simulink model "PistonControllerOff"  (R2013a)
settings: Solver=FixedStepDiscrete  StartTime=0.0  StopTime=75  FixedStep=0.001  RelTol=1e-3
InitFcn:
  | % PI gains
  | 
  | P1 = 15.0;
  | I1 = 100.0;
  | D1 = 10.0;
  | N1 = 10;
  | 
  | 
  | P2 =15.0 ;
  | I2 = 100.0;
  | D2 = 0.0;
  | N2 = 5;
  | 
  | P3 = 15.0;
  | I3 = 100.0;
  | D3 = 0.0;
  | N3 = 5;
  | 
  | P4 =15.0;
  | I4 = 100.0;
  | D4 =0.0;
  | N4 = 5;
  | 
  | P5 = 15.0;
  | I5 = 100.0;
  | D5 = 0.0;
  | N5 = 5;
  | 
  | P6 = 40.0;
  | I6 = 100.0;
  | D6 = 0.0;
  | N6 = 5.0;
  | 
  | P7 = 6.7;
  | I7 = 0.0;
  | D7 = 0.0;
  | N7 = 10.0;
  | 
  | %Max = Left = positive
  | 
  | offset = 1000;
  | 
  | max1 = 2300;
  | min1 = -2300;
  | 
  | max2 = 2500;
  | min2 = -2500;
  | 
  | max3 = 2600;
  | min3 = -2600;
  | 
  | max4 = 2600;
  | min4 = -2600;
  | 
  | max5 = 2600;
  | min5 = -2600;
  | 
  | max6 = 2400;
  | min6 = -2400;
  | 
  | 
  | max_posG = 1800;
undefined symbols (not defined in the file or in its folder): rtwindemocb_modeswitch, Serial_Port, Standard_Devices
libraries: rtwinlib x14, simulink x7
Description:
  | Packet Input/Output
  | 
  | This model shows how to transfer data through UDP
  | communication protocol using binary encoding. The model sends data
  | within one computer, from one UDP port to another. You can modify the
  | model to communicate between two computers by splitting this model
  | into its send and receive parts and running the models on two computers.
  | The yellow blocks are used to send the data, the blue blocks
  | are used to receive the data. Then, please enter the IP addresses of the two
  | computers into the appropriate fields in the Board Setup dialog.
  | 
  | How to run this model in Normal Mode:
  | 
  | 1) Double-click the orange button to switch to Normal Mode if needed.
  | 2) Start the real-time execution using Simulation->Run.
  | 
  | How to run this model in External Mode:
  | 
  | 1) Double-click the orange button to switch to External Mode if needed.
  | 2) Build the model using Code->C/C++ Code->Build Model.
  | 3) Connect to the real-time code using Simulation->Connect To Target.
  | 4) Start the real-time execution using Simulation->Run.
settings Model: SimulationMode=external  ExtModeTrigDuration=75001  Creator=The MathWorks Inc.  LastModifiedBy=drl
settings DataIOCC: SignalLoggingSaveFormat=ModelDataLogs
settings OptimizationCC: InlineParams=on  InlineInvariantSignals=on  EnhancedBackFolding=on  ExpressionDepthLimit=2147483647  InitFltsAndDblsToZero=on  EfficientFloat2IntCast=on  EfficientMapNaN2IntZero=off  SimCompilerOptimization=On
settings DebuggingCC: MultiTaskDSMMsg=warning  MultiTaskCondExecSysMsg=none  FcnCallInpInsideContextMsg=EnableAllAsWarning  StrictBusMsg=None
settings HardwareCC: ProdIntDivRoundTo=Zero  ProdEndianess=LittleEndian  ProdHWDeviceType=32-bit Real-Time Windows Target  TargetIntDivRoundTo=Zero  TargetEndianess=LittleEndian  TargetHWDeviceType=32-bit Real-Time Windows Target
settings ModelReferenceCC: UpdateModelReferenceTargets=IfOutOfDate
settings SFSimCC: SFSimEcho=off
settings RTWCC: SystemTargetFile=rtwin.tlc  TemplateMakefile=rtwin.tmf  Description=Real-Time Windows Target  ProcessScript=rtwin_make_rtw_hook  IncludeERTFirstTime=on  RTWCompilerOptimization=On
settings RTWinTargetCC: TargetLibSuffix=_rtwin.lib  TargetPreCompLibLocation=C:\Program Files\MATLAB\R2013a\toolbox\rtw\targets\rtwin\lib\win64  CodeReplacementLibrary=ANSI_C  RTWinDir=C:/PROGRA~1/MATLAB/R2013a/toolbox/rtw/targets/rtwin  TargetArch=win64

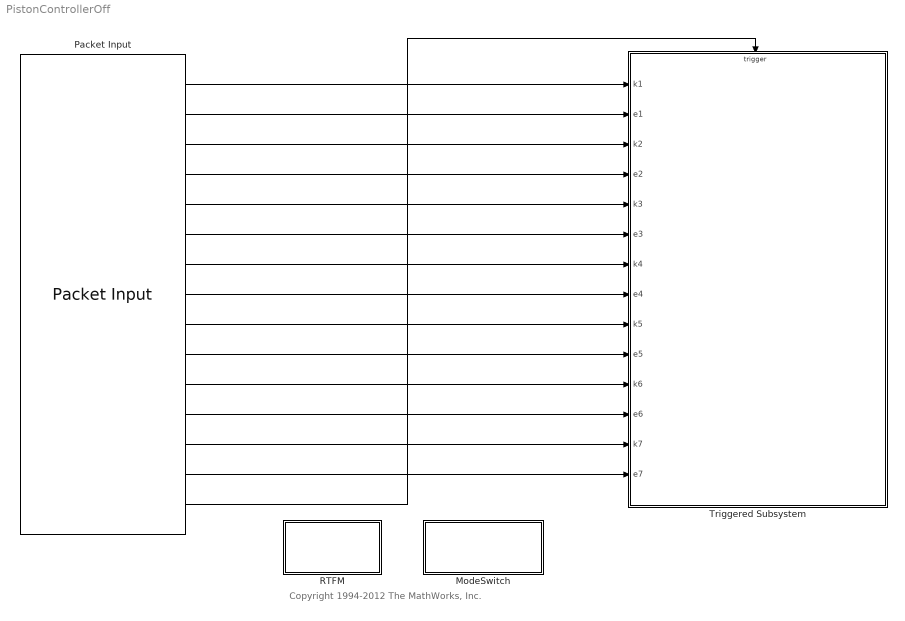
== system PistonControllerOff ==
  note: Copyright 1994-2012 The MathWorks, Inc.
  ModeSwitch : Subsystem  InitFcn=rtwindemocb_modeswitch('CheckKernel');  mask(Real-Time Windows Target Example Mode Switch){}
      settings: OpenFcn=rtwindemocb_modeswitch(gcbh);
      mask Display: disp('Switch To\nNormal Mode');
  Packet Input : rtwinlib/Packet Input  SampleTime=0.001  MaxMissedTicks=10000  ShowMissedTicks=off  YieldWhenWaiting=off  DrvName=Standard_Devices/Serial_Port  DrvAddress=39  DrvOptions=[57600 8 0 0 0 0 0 0]  PacketSize=14  DataTypes={'int8','int8','int8','int8','int8','int8','int8','int8','int8','int8','int8','int8','int8','int8'}  ShowReady=on  ShowError=off  PacketID=1  ByteOrder=1  ShowTimestamp=off
      settings: AttributesFormatString=Standard Devices\nSerial Port [27h]
  "RTFM " : Subsystem  mask(Real-Time Windows Target Example Info){}
      settings: OpenFcn=web(fullfile(fileparts(which(gcs)), 'html', [gcs '.html']), '-helpbrowser');
      mask Display: disp('Info')
  Triggered Subsystem : Subsystem  TreatAsAtomicUnit=on
  wires:
  Packet Input/10 -> Triggered Subsystem/10(e5)
  Packet Input/4 -> Triggered Subsystem/4(e2)
  Packet Input/12 -> Triggered Subsystem/12(e6)
  Packet Input/8 -> Triggered Subsystem/8(e4)
  Packet Input/9 -> Triggered Subsystem/9(k5)
  Packet Input/11 -> Triggered Subsystem/11(k6)
  Packet Input/5 -> Triggered Subsystem/5(k3)
  Packet Input/7 -> Triggered Subsystem/7(k4)
  Packet Input/6 -> Triggered Subsystem/6(e3)
  Packet Input/1 -> Triggered Subsystem/1(k1)
  Packet Input/3 -> Triggered Subsystem/3(k2)
  Packet Input/2 -> Triggered Subsystem/2(e1)
  Packet Input/13 -> Triggered Subsystem/13(k7)
  Packet Input/14 -> Triggered Subsystem/14(e7)
  Packet Input/15 -> Triggered Subsystem/Trigger

== system PistonControllerOff/ModeSwitch ==

== system PistonControllerOff/RTFM  ==

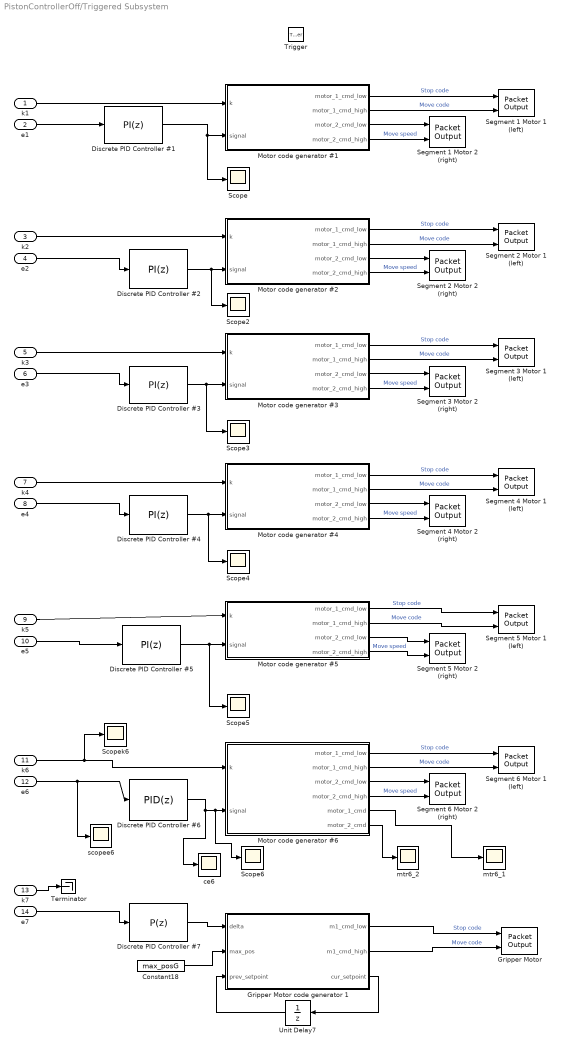
== system PistonControllerOff/Triggered Subsystem ==
  k1 : Inport
  e1 : Inport  Port=2
  k2 : Inport  Port=3
  e2 : Inport  Port=4
  k3 : Inport  Port=5
  e3 : Inport  Port=6
  k4 : Inport  Port=7
  e4 : Inport  Port=8
  k5 : Inport  Port=9
  e5 : Inport  Port=10
  k6 : Inport  Port=11
  e6 : Inport  Port=12
  k7 : Inport  Port=13
  e7 : Inport  Port=14
  Trigger : TriggerPort
  Constant18 : Constant  Value=max_posG
  Discrete PID Controller #1 : simulink/Continuous/PID Controller  Controller=PI  TimeDomain=Discrete-time  SampleTime=-1  IntegratorMethod=Forward Euler  FilterMethod=Forward Euler  Form=Parallel  P=P1  I=I1  D=D1  N=N1  InitialConditionSource=internal  InitialConditionForIntegrator=0  InitialConditionForFilter=0  ExternalReset=none  LimitOutput=on  UpperSaturationLimit=max1  LowerSaturationLimit=min1  LinearizeAsGain=off  AntiWindupMode=clamping  Kb=1  TrackingMode=off  Kt=10  RndMeth=Nearest  SaturateOnIntegerOverflow=on  PParamMin=[]  PParamMax=[]  PParamDataTypeStr=double  IParamMin=[]  IParamMax=[]  IParamDataTypeStr=double  DParamMin=[]  DParamMax=[]  DParamDataTypeStr=double  NParamMin=[]  NParamMax=[]  NParamDataTypeStr=double  KbParamMin=[]  KbParamMax=[]  KtParamMin=[]  KtParamMax=[]  KtParamDataTypeStr=double  POutMin=[]  POutMax=[]  POutDataTypeStr=double  IOutMin=[]  IOutMax=[]  IOutDataTypeStr=double  DOutMin=[]  DOutMax=[]  DOutDataTypeStr=double  NOutMin=[]  NOutMax=[]  NOutDataTypeStr=double  KbOutMin=[]  KbOutMax=[]  KtOutMin=[]  KtOutMax=[]  KtOutDataTypeStr=double  IntegratorOutMin=[]  IntegratorOutMax=[]  IntegratorOutDataTypeStr=double  FilterOutMin=[]  FilterOutMax=[]  FilterOutDataTypeStr=double  SumOutMin=[]  SumOutMax=[]  SumOutDataTypeStr=double  SumI1OutMin=[]  SumI1OutMax=[]  SumI1OutDataTypeStr=double  SumI2OutMin=[]  SumI2OutMax=[]  SumI3OutMin=[]  SumI3OutMax=[]  SumI3OutDataTypeStr=double  SumDOutMin=[]  SumDOutMax=[]  SumDOutDataTypeStr=double  SumAccumDataTypeStr=double  SumI1AccumDataTypeStr=double  SumI3AccumDataTypeStr=double  SumDAccumDataTypeStr=double  SaturationOutMin=[]  SaturationOutMax=[]  SaturationOutDataTypeStr=double  IntegratorContinuousStateAttributes=''  IntegratorStateMustResolveToSignalObject=off  IntegratorRTWStateStorageClass=Auto  FilterContinuousStateAttributes=''  FilterStateMustResolveToSignalObject=off  FilterRTWStateStorageClass=Auto
  Discrete PID Controller #2 : simulink/Continuous/PID Controller  Controller=PI  TimeDomain=Discrete-time  SampleTime=-1  IntegratorMethod=Forward Euler  FilterMethod=Forward Euler  Form=Parallel  P=P2  I=I2  D=D2  N=N2  InitialConditionSource=internal  InitialConditionForIntegrator=0  InitialConditionForFilter=0  ExternalReset=none  LimitOutput=on  UpperSaturationLimit=max2  LowerSaturationLimit=min2  LinearizeAsGain=off  AntiWindupMode=clamping  Kb=1  TrackingMode=off  Kt=10  RndMeth=Nearest  SaturateOnIntegerOverflow=on  PParamMin=[]  PParamMax=[]  PParamDataTypeStr=double  IParamMin=[]  IParamMax=[]  IParamDataTypeStr=double  DParamMin=[]  DParamMax=[]  DParamDataTypeStr=double  NParamMin=[]  NParamMax=[]  NParamDataTypeStr=double  KbParamMin=[]  KbParamMax=[]  KtParamMin=[]  KtParamMax=[]  KtParamDataTypeStr=double  POutMin=[]  POutMax=[]  POutDataTypeStr=double  IOutMin=[]  IOutMax=[]  IOutDataTypeStr=double  DOutMin=[]  DOutMax=[]  DOutDataTypeStr=double  NOutMin=[]  NOutMax=[]  NOutDataTypeStr=double  KbOutMin=[]  KbOutMax=[]  KtOutMin=[]  KtOutMax=[]  KtOutDataTypeStr=double  IntegratorOutMin=[]  IntegratorOutMax=[]  IntegratorOutDataTypeStr=double  FilterOutMin=[]  FilterOutMax=[]  FilterOutDataTypeStr=double  SumOutMin=[]  SumOutMax=[]  SumOutDataTypeStr=double  SumI1OutMin=[]  SumI1OutMax=[]  SumI1OutDataTypeStr=double  SumI2OutMin=[]  SumI2OutMax=[]  SumI3OutMin=[]  SumI3OutMax=[]  SumI3OutDataTypeStr=double  SumDOutMin=[]  SumDOutMax=[]  SumDOutDataTypeStr=double  SumAccumDataTypeStr=double  SumI1AccumDataTypeStr=double  SumI3AccumDataTypeStr=double  SumDAccumDataTypeStr=double  SaturationOutMin=[]  SaturationOutMax=[]  SaturationOutDataTypeStr=double  IntegratorContinuousStateAttributes=''  IntegratorStateMustResolveToSignalObject=off  IntegratorRTWStateStorageClass=Auto  FilterContinuousStateAttributes=''  FilterStateMustResolveToSignalObject=off  FilterRTWStateStorageClass=Auto
  Discrete PID Controller #3 : simulink/Continuous/PID Controller  Controller=PI  TimeDomain=Discrete-time  SampleTime=-1  IntegratorMethod=Forward Euler  FilterMethod=Forward Euler  Form=Parallel  P=P3  I=I3  D=D3  N=N3  InitialConditionSource=internal  InitialConditionForIntegrator=0  InitialConditionForFilter=0  ExternalReset=none  LimitOutput=on  UpperSaturationLimit=max3  LowerSaturationLimit=min3  LinearizeAsGain=off  AntiWindupMode=clamping  Kb=1  TrackingMode=off  Kt=10  RndMeth=Nearest  SaturateOnIntegerOverflow=on  PParamMin=[]  PParamMax=[]  PParamDataTypeStr=double  IParamMin=[]  IParamMax=[]  IParamDataTypeStr=double  DParamMin=[]  DParamMax=[]  DParamDataTypeStr=double  NParamMin=[]  NParamMax=[]  NParamDataTypeStr=double  KbParamMin=[]  KbParamMax=[]  KtParamMin=[]  KtParamMax=[]  KtParamDataTypeStr=double  POutMin=[]  POutMax=[]  POutDataTypeStr=double  IOutMin=[]  IOutMax=[]  IOutDataTypeStr=double  DOutMin=[]  DOutMax=[]  DOutDataTypeStr=double  NOutMin=[]  NOutMax=[]  NOutDataTypeStr=double  KbOutMin=[]  KbOutMax=[]  KtOutMin=[]  KtOutMax=[]  KtOutDataTypeStr=double  IntegratorOutMin=[]  IntegratorOutMax=[]  IntegratorOutDataTypeStr=double  FilterOutMin=[]  FilterOutMax=[]  FilterOutDataTypeStr=double  SumOutMin=[]  SumOutMax=[]  SumOutDataTypeStr=double  SumI1OutMin=[]  SumI1OutMax=[]  SumI1OutDataTypeStr=double  SumI2OutMin=[]  SumI2OutMax=[]  SumI3OutMin=[]  SumI3OutMax=[]  SumI3OutDataTypeStr=double  SumDOutMin=[]  SumDOutMax=[]  SumDOutDataTypeStr=double  SumAccumDataTypeStr=double  SumI1AccumDataTypeStr=double  SumI3AccumDataTypeStr=double  SumDAccumDataTypeStr=double  SaturationOutMin=[]  SaturationOutMax=[]  SaturationOutDataTypeStr=double  IntegratorContinuousStateAttributes=''  IntegratorStateMustResolveToSignalObject=off  IntegratorRTWStateStorageClass=Auto  FilterContinuousStateAttributes=''  FilterStateMustResolveToSignalObject=off  FilterRTWStateStorageClass=Auto
  Discrete PID Controller #4 : simulink/Continuous/PID Controller  Controller=PI  TimeDomain=Discrete-time  SampleTime=-1  IntegratorMethod=Forward Euler  FilterMethod=Forward Euler  Form=Parallel  P=P4  I=I4  D=D4  N=N4  InitialConditionSource=internal  InitialConditionForIntegrator=0  InitialConditionForFilter=0  ExternalReset=none  LimitOutput=on  UpperSaturationLimit=max4  LowerSaturationLimit=min4  LinearizeAsGain=off  AntiWindupMode=clamping  Kb=1  TrackingMode=off  Kt=10  RndMeth=Nearest  SaturateOnIntegerOverflow=on  PParamMin=[]  PParamMax=[]  PParamDataTypeStr=double  IParamMin=[]  IParamMax=[]  IParamDataTypeStr=double  DParamMin=[]  DParamMax=[]  DParamDataTypeStr=double  NParamMin=[]  NParamMax=[]  NParamDataTypeStr=double  KbParamMin=[]  KbParamMax=[]  KtParamMin=[]  KtParamMax=[]  KtParamDataTypeStr=double  POutMin=[]  POutMax=[]  POutDataTypeStr=double  IOutMin=[]  IOutMax=[]  IOutDataTypeStr=double  DOutMin=[]  DOutMax=[]  DOutDataTypeStr=double  NOutMin=[]  NOutMax=[]  NOutDataTypeStr=double  KbOutMin=[]  KbOutMax=[]  KtOutMin=[]  KtOutMax=[]  KtOutDataTypeStr=double  IntegratorOutMin=[]  IntegratorOutMax=[]  IntegratorOutDataTypeStr=double  FilterOutMin=[]  FilterOutMax=[]  FilterOutDataTypeStr=double  SumOutMin=[]  SumOutMax=[]  SumOutDataTypeStr=double  SumI1OutMin=[]  SumI1OutMax=[]  SumI1OutDataTypeStr=double  SumI2OutMin=[]  SumI2OutMax=[]  SumI3OutMin=[]  SumI3OutMax=[]  SumI3OutDataTypeStr=double  SumDOutMin=[]  SumDOutMax=[]  SumDOutDataTypeStr=double  SumAccumDataTypeStr=double  SumI1AccumDataTypeStr=double  SumI3AccumDataTypeStr=double  SumDAccumDataTypeStr=double  SaturationOutMin=[]  SaturationOutMax=[]  SaturationOutDataTypeStr=double  IntegratorContinuousStateAttributes=''  IntegratorStateMustResolveToSignalObject=off  IntegratorRTWStateStorageClass=Auto  FilterContinuousStateAttributes=''  FilterStateMustResolveToSignalObject=off  FilterRTWStateStorageClass=Auto
  Discrete PID Controller #5 : simulink/Continuous/PID Controller  Controller=PI  TimeDomain=Discrete-time  SampleTime=-1  IntegratorMethod=Forward Euler  FilterMethod=Forward Euler  Form=Parallel  P=P3  I=I3  D=D3  N=N3  InitialConditionSource=internal  InitialConditionForIntegrator=0  InitialConditionForFilter=0  ExternalReset=none  LimitOutput=on  UpperSaturationLimit=max5  LowerSaturationLimit=min5  LinearizeAsGain=off  AntiWindupMode=clamping  Kb=1  TrackingMode=off  Kt=10  RndMeth=Nearest  SaturateOnIntegerOverflow=on  PParamMin=[]  PParamMax=[]  PParamDataTypeStr=double  IParamMin=[]  IParamMax=[]  IParamDataTypeStr=double  DParamMin=[]  DParamMax=[]  DParamDataTypeStr=double  NParamMin=[]  NParamMax=[]  NParamDataTypeStr=double  KbParamMin=[]  KbParamMax=[]  KtParamMin=[]  KtParamMax=[]  KtParamDataTypeStr=double  POutMin=[]  POutMax=[]  POutDataTypeStr=double  IOutMin=[]  IOutMax=[]  IOutDataTypeStr=double  DOutMin=[]  DOutMax=[]  DOutDataTypeStr=double  NOutMin=[]  NOutMax=[]  NOutDataTypeStr=double  KbOutMin=[]  KbOutMax=[]  KtOutMin=[]  KtOutMax=[]  KtOutDataTypeStr=double  IntegratorOutMin=[]  IntegratorOutMax=[]  IntegratorOutDataTypeStr=double  FilterOutMin=[]  FilterOutMax=[]  FilterOutDataTypeStr=double  SumOutMin=[]  SumOutMax=[]  SumOutDataTypeStr=double  SumI1OutMin=[]  SumI1OutMax=[]  SumI1OutDataTypeStr=double  SumI2OutMin=[]  SumI2OutMax=[]  SumI3OutMin=[]  SumI3OutMax=[]  SumI3OutDataTypeStr=double  SumDOutMin=[]  SumDOutMax=[]  SumDOutDataTypeStr=double  SumAccumDataTypeStr=double  SumI1AccumDataTypeStr=double  SumI3AccumDataTypeStr=double  SumDAccumDataTypeStr=double  SaturationOutMin=[]  SaturationOutMax=[]  SaturationOutDataTypeStr=double  IntegratorContinuousStateAttributes=''  IntegratorStateMustResolveToSignalObject=off  IntegratorRTWStateStorageClass=Auto  FilterContinuousStateAttributes=''  FilterStateMustResolveToSignalObject=off  FilterRTWStateStorageClass=Auto
  Discrete PID Controller #6 : simulink/Continuous/PID Controller  Controller=PID  TimeDomain=Discrete-time  SampleTime=-1  IntegratorMethod=Forward Euler  FilterMethod=Forward Euler  Form=Parallel  P=P6  I=I6  D=D6  N=N6  InitialConditionSource=internal  InitialConditionForIntegrator=0  InitialConditionForFilter=0  ExternalReset=none  LimitOutput=on  UpperSaturationLimit=max6  LowerSaturationLimit=min6  LinearizeAsGain=off  AntiWindupMode=clamping  Kb=1  TrackingMode=off  Kt=10  RndMeth=Nearest  SaturateOnIntegerOverflow=on  PParamMin=[]  PParamMax=[]  PParamDataTypeStr=double  IParamMin=[]  IParamMax=[]  IParamDataTypeStr=double  DParamMin=[]  DParamMax=[]  DParamDataTypeStr=double  NParamMin=[]  NParamMax=[]  NParamDataTypeStr=double  KbParamMin=[]  KbParamMax=[]  KtParamMin=[]  KtParamMax=[]  KtParamDataTypeStr=double  POutMin=[]  POutMax=[]  POutDataTypeStr=double  IOutMin=[]  IOutMax=[]  IOutDataTypeStr=double  DOutMin=[]  DOutMax=[]  DOutDataTypeStr=double  NOutMin=[]  NOutMax=[]  NOutDataTypeStr=double  KbOutMin=[]  KbOutMax=[]  KtOutMin=[]  KtOutMax=[]  KtOutDataTypeStr=double  IntegratorOutMin=[]  IntegratorOutMax=[]  IntegratorOutDataTypeStr=double  FilterOutMin=[]  FilterOutMax=[]  FilterOutDataTypeStr=double  SumOutMin=[]  SumOutMax=[]  SumOutDataTypeStr=double  SumI1OutMin=[]  SumI1OutMax=[]  SumI1OutDataTypeStr=double  SumI2OutMin=[]  SumI2OutMax=[]  SumI3OutMin=[]  SumI3OutMax=[]  SumI3OutDataTypeStr=double  SumDOutMin=[]  SumDOutMax=[]  SumDOutDataTypeStr=double  SumAccumDataTypeStr=double  SumI1AccumDataTypeStr=double  SumI3AccumDataTypeStr=double  SumDAccumDataTypeStr=double  SaturationOutMin=[]  SaturationOutMax=[]  SaturationOutDataTypeStr=double  IntegratorContinuousStateAttributes=''  IntegratorStateMustResolveToSignalObject=off  IntegratorRTWStateStorageClass=Auto  FilterContinuousStateAttributes=''  FilterStateMustResolveToSignalObject=off  FilterRTWStateStorageClass=Auto
  Discrete PID Controller #7 : simulink/Continuous/PID Controller  Controller=P  TimeDomain=Discrete-time  SampleTime=-1  IntegratorMethod=Forward Euler  FilterMethod=Forward Euler  Form=Parallel  P=P7  I=I7  D=D7  N=N7  InitialConditionSource=internal  InitialConditionForIntegrator=0  InitialConditionForFilter=0  ExternalReset=none  LimitOutput=on  UpperSaturationLimit=800  LowerSaturationLimit=-800  LinearizeAsGain=off  AntiWindupMode=clamping  Kb=1  TrackingMode=off  Kt=10  RndMeth=Nearest  SaturateOnIntegerOverflow=on  PParamMin=[]  PParamMax=[]  PParamDataTypeStr=double  IParamMin=[]  IParamMax=[]  IParamDataTypeStr=double  DParamMin=[]  DParamMax=[]  DParamDataTypeStr=double  NParamMin=[]  NParamMax=[]  NParamDataTypeStr=double  KbParamMin=[]  KbParamMax=[]  KtParamMin=[]  KtParamMax=[]  KtParamDataTypeStr=double  POutMin=[]  POutMax=[]  POutDataTypeStr=double  IOutMin=[]  IOutMax=[]  IOutDataTypeStr=double  DOutMin=[]  DOutMax=[]  DOutDataTypeStr=double  NOutMin=[]  NOutMax=[]  NOutDataTypeStr=double  KbOutMin=[]  KbOutMax=[]  KtOutMin=[]  KtOutMax=[]  KtOutDataTypeStr=double  IntegratorOutMin=[]  IntegratorOutMax=[]  IntegratorOutDataTypeStr=double  FilterOutMin=[]  FilterOutMax=[]  FilterOutDataTypeStr=double  SumOutMin=[]  SumOutMax=[]  SumOutDataTypeStr=double  SumI1OutMin=[]  SumI1OutMax=[]  SumI1OutDataTypeStr=double  SumI2OutMin=[]  SumI2OutMax=[]  SumI3OutMin=[]  SumI3OutMax=[]  SumI3OutDataTypeStr=double  SumDOutMin=[]  SumDOutMax=[]  SumDOutDataTypeStr=double  SumAccumDataTypeStr=double  SumI1AccumDataTypeStr=double  SumI3AccumDataTypeStr=double  SumDAccumDataTypeStr=double  SaturationOutMin=[]  SaturationOutMax=[]  SaturationOutDataTypeStr=double  IntegratorContinuousStateAttributes=''  IntegratorStateMustResolveToSignalObject=off  IntegratorRTWStateStorageClass=Auto  FilterContinuousStateAttributes=''  FilterStateMustResolveToSignalObject=off  FilterRTWStateStorageClass=Auto
  Gripper Motor : rtwinlib/Packet Output  SampleTime=-1  MaxMissedTicks=10  ShowMissedTicks=off  YieldWhenWaiting=off  DrvName=Standard_Devices/Serial_Port  DrvAddress=68  DrvOptions=[57600 8 0 0 0 0 0 0]  PacketSize=2  DataTypes={'uint8','uint8'}  ShowReady=off  ShowError=off  PacketID=1  ByteOrder=1  InitialValue=[192, 0]  FinalValue=[192, 0]
      settings: AttributesFormatString=Standard Devices\nSerial Port [44h]
  Gripper Motor code generator 1 : MATLAB Function  TreatAsAtomicUnit=on
  Motor code generator #1 : MATLAB Function  TreatAsAtomicUnit=on
  Motor code generator #2 : MATLAB Function  TreatAsAtomicUnit=on
  Motor code generator #3 : MATLAB Function  TreatAsAtomicUnit=on
  Motor code generator #4 : MATLAB Function  TreatAsAtomicUnit=on
  Motor code generator #5 : MATLAB Function  TreatAsAtomicUnit=on
  Motor code generator #6 : MATLAB Function  TreatAsAtomicUnit=on
  Scope{,2..6} (6 alike) : Scope
      Scope settings: SaveName=zoffset1
      Scope2 settings: SaveName=zoffset2
      Scope3 settings: SaveName=zoffset3
      Scope4 settings: SaveName=zoffset4
      Scope5 settings: SaveName=zoffset5
      Scope6 settings: SaveName=zoffset6
  "Scopek6 " : Scope
      settings: ShowLegends=on  YMin=-35  YMax=35  SaveName=k6  MaxDataPoints=30000
  Segment 1 Motor 1 (left) : rtwinlib/Packet Output  SampleTime=-1  MaxMissedTicks=10  ShowMissedTicks=off  YieldWhenWaiting=off  DrvName=Standard_Devices/Serial_Port  DrvAddress=19  DrvOptions=[57600 8 0 0 0 0 0 0]  PacketSize=2  DataTypes={'uint8','uint8'}  ShowReady=off  ShowError=off  PacketID=1  ByteOrder=1  InitialValue=[216, 43]  FinalValue=[200, 31]
      settings: AttributesFormatString=Standard Devices\nSerial Port [13h]
  Segment 1 Motor 2 (right) : rtwinlib/Packet Output  SampleTime=-1  MaxMissedTicks=10  ShowMissedTicks=off  YieldWhenWaiting=off  DrvName=Standard_Devices/Serial_Port  DrvAddress=22  DrvOptions=[57600 8 0 0 0 0 0 0]  PacketSize=2  DataTypes={'uint8','uint8'}  ShowReady=off  ShowError=off  PacketID=1  ByteOrder=1  InitialValue=[216, 43]  FinalValue=[200, 31]
      settings: AttributesFormatString=Standard Devices\nSerial Port [16h]
  Segment 2 Motor 1 (left) : rtwinlib/Packet Output  SampleTime=-1  MaxMissedTicks=10  ShowMissedTicks=off  YieldWhenWaiting=off  DrvName=Standard_Devices/Serial_Port  DrvAddress=23  DrvOptions=[57600 8 0 0 0 0 0 0]  PacketSize=2  DataTypes={'uint8','uint8'}  ShowReady=off  ShowError=off  PacketID=1  ByteOrder=1  InitialValue=[216, 43]  FinalValue=[200, 31]
      settings: AttributesFormatString=Standard Devices\nSerial Port [17h]
  Segment 2 Motor 2 (right) : rtwinlib/Packet Output  SampleTime=-1  MaxMissedTicks=10  ShowMissedTicks=off  YieldWhenWaiting=off  DrvName=Standard_Devices/Serial_Port  DrvAddress=25  DrvOptions=[57600 8 0 0 0 0 0 0]  PacketSize=2  DataTypes={'uint8','uint8'}  ShowReady=off  ShowError=off  PacketID=1  ByteOrder=1  InitialValue=[216, 43]  FinalValue=[200, 31]
      settings: AttributesFormatString=Standard Devices\nSerial Port [19h]
  Segment 3 Motor 1 (left) : rtwinlib/Packet Output  SampleTime=-1  MaxMissedTicks=10  ShowMissedTicks=off  YieldWhenWaiting=off  DrvName=Standard_Devices/Serial_Port  DrvAddress=17  DrvOptions=[57600 8 0 0 0 0 0 0]  PacketSize=2  DataTypes={'uint8','uint8'}  ShowReady=off  ShowError=off  PacketID=1  ByteOrder=1  InitialValue=[212, 40]  FinalValue=[212, 40]
      settings: AttributesFormatString=Standard Devices\nSerial Port [11h]
  Segment 3 Motor 2 (right) : rtwinlib/Packet Output  SampleTime=-1  MaxMissedTicks=10  ShowMissedTicks=off  YieldWhenWaiting=off  DrvName=Standard_Devices/Serial_Port  DrvAddress=16  DrvOptions=[57600 8 0 0 0 0 0 0]  PacketSize=2  DataTypes={'uint8','uint8'}  ShowReady=off  ShowError=off  PacketID=1  ByteOrder=1  InitialValue=[212, 40]  FinalValue=[200, 31]
      settings: AttributesFormatString=Standard Devices\nSerial Port [10h]
  Segment 4 Motor 1 (left) : rtwinlib/Packet Output  SampleTime=-1  MaxMissedTicks=10  ShowMissedTicks=off  YieldWhenWaiting=off  DrvName=Standard_Devices/Serial_Port  DrvAddress=27  DrvOptions=[57600 8 0 0 0 0 0 0]  PacketSize=2  DataTypes={'uint8','uint8'}  ShowReady=off  ShowError=off  PacketID=1  ByteOrder=1  InitialValue=[212, 40]  FinalValue=[200, 31]
      settings: AttributesFormatString=Standard Devices\nSerial Port [1Bh]
  Segment 4 Motor 2 (right) : rtwinlib/Packet Output  SampleTime=-1  MaxMissedTicks=10  ShowMissedTicks=off  YieldWhenWaiting=off  DrvName=Standard_Devices/Serial_Port  DrvAddress=29  DrvOptions=[57600 8 0 0 0 0 0 0]  PacketSize=2  DataTypes={'uint8','uint8'}  ShowReady=off  ShowError=off  PacketID=1  ByteOrder=1  InitialValue=[212, 40]  FinalValue=[200, 31]
      settings: AttributesFormatString=Standard Devices\nSerial Port [1Dh]
  Segment 5 Motor 1 (left) : rtwinlib/Packet Output  SampleTime=-1  MaxMissedTicks=10  ShowMissedTicks=off  YieldWhenWaiting=off  DrvName=Standard_Devices/Serial_Port  DrvAddress=31  DrvOptions=[57600 8 0 0 0 0 0 0]  PacketSize=2  DataTypes={'uint8','uint8'}  ShowReady=off  ShowError=off  PacketID=1  ByteOrder=1  InitialValue=[212, 40]  FinalValue=[200, 31]
      settings: AttributesFormatString=Standard Devices\nSerial Port [1Fh]
  Segment 5 Motor 2 (right) : rtwinlib/Packet Output  SampleTime=-1  MaxMissedTicks=10  ShowMissedTicks=off  YieldWhenWaiting=off  DrvName=Standard_Devices/Serial_Port  DrvAddress=34  DrvOptions=[57600 8 0 0 0 0 0 0]  PacketSize=2  DataTypes={'uint8','uint8'}  ShowReady=off  ShowError=off  PacketID=1  ByteOrder=1  InitialValue=[212, 40]  FinalValue=[200, 31]
      settings: AttributesFormatString=Standard Devices\nSerial Port [22h]
  Segment 6 Motor 1 (left) : rtwinlib/Packet Output  SampleTime=-1  MaxMissedTicks=10  ShowMissedTicks=off  YieldWhenWaiting=off  DrvName=Standard_Devices/Serial_Port  DrvAddress=35  DrvOptions=[57600 8 0 0 0 0 0 0]  PacketSize=2  DataTypes={'uint8','uint8'}  ShowReady=off  ShowError=off  PacketID=1  ByteOrder=1  InitialValue=[212, 40]  FinalValue=[200, 31]
      settings: AttributesFormatString=Standard Devices\nSerial Port [23h]
  Segment 6 Motor 2 (right) : rtwinlib/Packet Output  SampleTime=-1  MaxMissedTicks=10  ShowMissedTicks=off  YieldWhenWaiting=off  DrvName=Standard_Devices/Serial_Port  DrvAddress=38  DrvOptions=[57600 8 0 0 0 0 0 0]  PacketSize=2  DataTypes={'uint8','uint8'}  ShowReady=off  ShowError=off  PacketID=1  ByteOrder=1  InitialValue=[212, 40]  FinalValue=[200, 31]
      settings: AttributesFormatString=Standard Devices\nSerial Port [26h]
  Terminator : Terminator
  Unit Delay7 : UnitDelay  SampleTime=-1
  ce6 : Scope
      settings: ShowLegends=on  YMin=-35  YMax=35  SaveName=ce6  MaxDataPoints=30000
  mtr6_1 : Scope
      settings: ShowLegends=on  YMin=-35  YMax=35  SaveName=mtr6_1  MaxDataPoints=30000
  mtr6_2 : Scope
      settings: ShowLegends=on  YMin=-35  YMax=35  SaveName=mtr6_2  MaxDataPoints=30000
  scopee6 : Scope
      settings: ShowLegends=on  YMin=-35  YMax=35  SaveName=e6  MaxDataPoints=30000
  wires:
  e3/1 -> Discrete PID Controller #3/1
  Discrete PID Controller #3/1 -> Scope3/1, Motor code generator #3/2(signal)
  k3/1 -> Motor code generator #3/1(k)
  Motor code generator #3/1(motor_1_cmd_low) -> Segment 3 Motor 1 (left)/1  "Stop code"
  Motor code generator #3/2(motor_1_cmd_high) -> Segment 3 Motor 1 (left)/2  "Move code"
  Motor code generator #3/3(motor_2_cmd_low) -> Segment 3 Motor 2 (right)/1
  Motor code generator #3/4(motor_2_cmd_high) -> Segment 3 Motor 2 (right)/2  "Move speed"
  Discrete PID Controller #1/1 -> Scope/1, Motor code generator #1/2(signal)
  k1/1 -> Motor code generator #1/1(k)
  Motor code generator #1/1(motor_1_cmd_low) -> Segment 1 Motor 1 (left)/1  "Stop code"
  Motor code generator #1/2(motor_1_cmd_high) -> Segment 1 Motor 1 (left)/2  "Move code"
  Motor code generator #1/3(motor_2_cmd_low) -> Segment 1 Motor 2 (right)/1
  Motor code generator #1/4(motor_2_cmd_high) -> Segment 1 Motor 2 (right)/2  "Move speed"
  e1/1 -> Discrete PID Controller #1/1
  Discrete PID Controller #2/1 -> Scope2/1, Motor code generator #2/2(signal)
  k2/1 -> Motor code generator #2/1(k)
  Motor code generator #2/1(motor_1_cmd_low) -> Segment 2 Motor 1 (left)/1  "Stop code"
  Motor code generator #2/2(motor_1_cmd_high) -> Segment 2 Motor 1 (left)/2  "Move code"
  Motor code generator #2/3(motor_2_cmd_low) -> Segment 2 Motor 2 (right)/1
  Motor code generator #2/4(motor_2_cmd_high) -> Segment 2 Motor 2 (right)/2  "Move speed"
  e2/1 -> Discrete PID Controller #2/1
  Discrete PID Controller #4/1 -> Scope4/1, Motor code generator #4/2(signal)
  k4/1 -> Motor code generator #4/1(k)
  Motor code generator #4/1(motor_1_cmd_low) -> Segment 4 Motor 1 (left)/1  "Stop code"
  Motor code generator #4/2(motor_1_cmd_high) -> Segment 4 Motor 1 (left)/2  "Move code"
  Motor code generator #4/3(motor_2_cmd_low) -> Segment 4 Motor 2 (right)/1
  Motor code generator #4/4(motor_2_cmd_high) -> Segment 4 Motor 2 (right)/2  "Move speed"
  e4/1 -> Discrete PID Controller #4/1
  e5/1 -> Discrete PID Controller #5/1
  Discrete PID Controller #5/1 -> Scope5/1, Motor code generator #5/2(signal)
  k5/1 -> Motor code generator #5/1(k)
  Motor code generator #5/1(motor_1_cmd_low) -> Segment 5 Motor 1 (left)/1  "Stop code"
  Motor code generator #5/2(motor_1_cmd_high) -> Segment 5 Motor 1 (left)/2  "Move code"
  Motor code generator #5/3(motor_2_cmd_low) -> Segment 5 Motor 2 (right)/1
  Motor code generator #5/4(motor_2_cmd_high) -> Segment 5 Motor 2 (right)/2  "Move speed"
  e6/1 -> scopee6/1, Discrete PID Controller #6/1
  Discrete PID Controller #6/1 -> ce6/1, Scope6/1, Motor code generator #6/2(signal)
  k6/1 -> "Scopek6 "/1, Motor code generator #6/1(k)
  Motor code generator #6/1(motor_1_cmd_low) -> Segment 6 Motor 1 (left)/1  "Stop code"
  Motor code generator #6/2(motor_1_cmd_high) -> Segment 6 Motor 1 (left)/2  "Move code"
  Motor code generator #6/3(motor_2_cmd_low) -> Segment 6 Motor 2 (right)/1
  Motor code generator #6/4(motor_2_cmd_high) -> Segment 6 Motor 2 (right)/2  "Move speed"
  e7/1 -> Discrete PID Controller #7/1
  Gripper Motor code generator 1/1(m1_cmd_low) -> Gripper Motor/1  "Stop code"
  Gripper Motor code generator 1/2(m1_cmd_high) -> Gripper Motor/2  "Move code"
  Motor code generator #6/6(motor_2_cmd) -> mtr6_2/1
  Motor code generator #6/5(motor_1_cmd) -> mtr6_1/1
  Constant18/1 -> Gripper Motor code generator 1/2(max_pos)
  Gripper Motor code generator 1/3(cur_setpoint) -> Unit Delay7/1
  Unit Delay7/1 -> Gripper Motor code generator 1/3(prev_setpoint)
  Discrete PID Controller #7/1 -> Gripper Motor code generator 1/1(delta)
  k7/1 -> Terminator/1

== matlab function PistonControllerOff/Triggered Subsystem/Motor code generator #1 ==
  data: motor_1_cmd_low output; k input; motor_1_cmd_high output; motor_2_cmd_low output; signal input; motor_2_cmd_high output
function [motor_1_cmd_low, motor_1_cmd_high, motor_2_cmd_low, motor_2_cmd_high] = code_gen(k, signal)

zero_offset = 0.0;
signal = signal + zero_offset;
offset = uint16(1400);

position_setpoint = uint16(abs(signal));

if(signal <= 0.0)
    motor_2_cmd = offset;
    motor_1_cmd = offset + position_setpoint;
else
    motor_1_cmd = offset;
    motor_2_cmd = offset + position_setpoint;
end

% OLD CODE
% if (k == 1)
%     if(signal <= 0.0)
%         motor_2_cmd = offset;
%         motor_1_cmd = offset + position_setpoint;
%     else
%         motor_1_cmd = offset;
%         motor_2_cmd = offset + position_setpoint;
%     end
%     
% else
%     if(signal >= 0.0)
%         motor_1_cmd = offset;
%         motor_2_cmd = offset + position_setpoint;
%     else
%         motor_2_cmd = offset;
%         motor_1_cmd = offset + position_setpoint;
%     end
% end

%% Prepare motor output

motor_1_cmd_low = uint8(uint16(192) + bitand(motor_1_cmd, uint16(31)));
motor_1_cmd_high = uint8(bitand(bitshift(motor_1_cmd, -5), uint16(127)));

motor_2_cmd_low = uint8(uint16(192) + bitand(motor_2_cmd, uint16(31)));
motor_2_cmd_high = uint8(bitand(bitshift(motor_2_cmd, -5), uint16(127)));

== matlab function PistonControllerOff/Triggered Subsystem/Motor code generator #2 ==
  data: motor_1_cmd_low output; k input; motor_1_cmd_high output; motor_2_cmd_low output; signal input; motor_2_cmd_high output
function [motor_1_cmd_low, motor_1_cmd_high, motor_2_cmd_low, motor_2_cmd_high] = code_gen(k, signal)

zero_offset = 0;
signal = signal + zero_offset;

offset = uint16(1400);

position_setpoint = uint16(abs(signal));

if(signal <= 0.0)
    motor_2_cmd = offset;
    motor_1_cmd = offset + position_setpoint;
else
    motor_1_cmd = offset;
    motor_2_cmd = offset + position_setpoint;
end

% OLD CODE
% if (k == 1)
%     if(signal <= 0.0)
%         motor_2_cmd = offset;
%         motor_1_cmd = offset + position_setpoint;
%     else
%         motor_1_cmd = offset;
%         motor_2_cmd = offset + position_setpoint;
%     end
%     
% else
%     if(signal >= 0.0)
%         motor_1_cmd = offset;
%         motor_2_cmd = offset + position_setpoint;
%     else
%         motor_2_cmd = offset;
%         motor_1_cmd = offset + position_setpoint;
%     end
% end

%% Prepare motor output

motor_1_cmd_low = uint8(uint16(192) + bitand(motor_1_cmd, uint16(31)));
motor_1_cmd_high = uint8(bitand(bitshift(motor_1_cmd, -5), uint16(127)));

motor_2_cmd_low = uint8(uint16(192) + bitand(motor_2_cmd, uint16(31)));
motor_2_cmd_high = uint8(bitand(bitshift(motor_2_cmd, -5), uint16(127)));

== matlab function PistonControllerOff/Triggered Subsystem/Motor code generator #4 ==
  data: motor_1_cmd_low output; k input; motor_1_cmd_high output; motor_2_cmd_low output; signal input; motor_2_cmd_high output
function [motor_1_cmd_low, motor_1_cmd_high, motor_2_cmd_low, motor_2_cmd_high] = code_gen(k, signal)

zero_offset = 0;
signal = signal + zero_offset;

offset = uint16(1300);

position_setpoint = uint16(abs(signal));

if(signal <= 0.0)
    motor_2_cmd = offset;
    motor_1_cmd = offset + position_setpoint;
else
    motor_1_cmd = offset;
    motor_2_cmd = offset + position_setpoint;
end

% OLD CODE
% if (k == 1)
%     if(signal <= 0.0)
%         motor_2_cmd = offset;
%         motor_1_cmd = offset + position_setpoint;
%     else
%         motor_1_cmd = offset;
%         motor_2_cmd = offset + position_setpoint;
%     end
%     
% else
%     if(signal >= 0.0)
%         motor_1_cmd = offset;
%         motor_2_cmd = offset + position_setpoint;
%     else
%         motor_2_cmd = offset;
%         motor_1_cmd = offset + position_setpoint;
%     end
% end

%% Prepare motor output

motor_1_cmd_low = uint8(uint16(192) + bitand(motor_1_cmd, uint16(31)));
motor_1_cmd_high = uint8(bitand(bitshift(motor_1_cmd, -5), uint16(127)));

motor_2_cmd_low = uint8(uint16(192) + bitand(motor_2_cmd, uint16(31)));
motor_2_cmd_high = uint8(bitand(bitshift(motor_2_cmd, -5), uint16(127)));

== matlab function PistonControllerOff/Triggered Subsystem/Motor code generator #3 ==
  data: motor_1_cmd_low output; k input; motor_1_cmd_high output; motor_2_cmd_low output; signal input; motor_2_cmd_high output
function [motor_1_cmd_low, motor_1_cmd_high, motor_2_cmd_low, motor_2_cmd_high] = code_gen(k, signal)

zero_offset = 0;
signal = signal + zero_offset;

offset = uint16(1300);

position_setpoint = uint16(abs(signal));

if(signal <= 0.0)
    motor_2_cmd = offset;
    motor_1_cmd = offset + position_setpoint;
else
    motor_1_cmd = offset;
    motor_2_cmd = offset + position_setpoint;
end

% OLD CODE
% if (k == 1)
%     if(signal <= 0.0)
%         motor_2_cmd = offset;
%         motor_1_cmd = offset + position_setpoint;
%     else
%         motor_1_cmd = offset;
%         motor_2_cmd = offset + position_setpoint;
%     end
%     
% else
%     if(signal >= 0.0)
%         motor_1_cmd = offset;
%         motor_2_cmd = offset + position_setpoint;
%     else
%         motor_2_cmd = offset;
%         motor_1_cmd = offset + position_setpoint;
%     end
% end

%% Prepare motor output

motor_1_cmd_low = uint8(uint16(192) + bitand(motor_1_cmd, uint16(31)));
motor_1_cmd_high = uint8(bitand(bitshift(motor_1_cmd, -5), uint16(127)));

motor_2_cmd_low = uint8(uint16(192) + bitand(motor_2_cmd, uint16(31)));
motor_2_cmd_high = uint8(bitand(bitshift(motor_2_cmd, -5), uint16(127)));

== matlab function PistonControllerOff/Triggered Subsystem/Motor code generator #5 ==
  data: motor_1_cmd_low output; k input; motor_1_cmd_high output; motor_2_cmd_low output; signal input; motor_2_cmd_high output
function [motor_1_cmd_low, motor_1_cmd_high, motor_2_cmd_low, motor_2_cmd_high] = code_gen(k, signal)

zero_offset = 0;
signal = signal + zero_offset;

offset = uint16(1300);

position_setpoint = uint16(abs(signal));

if(signal <= 0.0)
    motor_2_cmd = offset;
    motor_1_cmd = offset + position_setpoint;
else
    motor_1_cmd = offset;
    motor_2_cmd = offset + position_setpoint;
end

% OLD CODE
% if (k == 1)
%     if(signal <= 0.0)
%         motor_2_cmd = offset;
%         motor_1_cmd = offset + position_setpoint;
%     else
%         motor_1_cmd = offset;
%         motor_2_cmd = offset + position_setpoint;
%     end
%     
% else
%     if(signal >= 0.0)
%         motor_1_cmd = offset;
%         motor_2_cmd = offset + position_setpoint;
%     else
%         motor_2_cmd = offset;
%         motor_1_cmd = offset + position_setpoint;
%     end
% end

%% Prepare motor output

motor_1_cmd_low = uint8(uint16(192) + bitand(motor_1_cmd, uint16(31)));
motor_1_cmd_high = uint8(bitand(bitshift(motor_1_cmd, -5), uint16(127)));

motor_2_cmd_low = uint8(uint16(192) + bitand(motor_2_cmd, uint16(31)));
motor_2_cmd_high = uint8(bitand(bitshift(motor_2_cmd, -5), uint16(127)));

== matlab function PistonControllerOff/Triggered Subsystem/Motor code generator #6 ==
  data: motor_1_cmd_low output; k input; motor_1_cmd_high output; motor_2_cmd_low output; signal input; motor_2_cmd_high output; motor_1_cmd output; motor_2_cmd output
function [motor_1_cmd_low, motor_1_cmd_high, motor_2_cmd_low, motor_2_cmd_high, motor_1_cmd, motor_2_cmd] = code_gen(k, signal)

zero_offset = 0;
signal = signal + zero_offset;

offset = uint16(1300);

position_setpoint = uint16(abs(signal));

if(signal <= 0.0)
    motor_2_cmd = offset;
    motor_1_cmd = offset + position_setpoint;
else
    motor_1_cmd = offset;
    motor_2_cmd = offset + position_setpoint;
end

% OLD CODE
% if (k == 1)
%     if(signal <= 0.0)
%         motor_2_cmd = offset;
%         motor_1_cmd = offset + position_setpoint;
%     else
%         motor_1_cmd = offset;
%         motor_2_cmd = offset + position_setpoint;
%     end
%     
% else
%     if(signal >= 0.0)
%         motor_1_cmd = offset;
%         motor_2_cmd = offset + position_setpoint;
%     else
%         motor_2_cmd = offset;
%         motor_1_cmd = offset + position_setpoint;
%     end
% end

%% Prepare motor output

motor_1_cmd_low = uint8(uint16(192) + bitand(motor_1_cmd, uint16(31)));
motor_1_cmd_high = uint8(bitand(bitshift(motor_1_cmd, -5), uint16(127)));

motor_2_cmd_low = uint8(uint16(192) + bitand(motor_2_cmd, uint16(31)));
motor_2_cmd_high = uint8(bitand(bitshift(motor_2_cmd, -5), uint16(127)));

== matlab function PistonControllerOff/Triggered Subsystem/Gripper Motor code generator 1 ==
  data: m1_cmd_low output; delta input; m1_cmd_high output; max_pos input; prev_setpoint input; cur_setpoint output
function [m1_cmd_low, m1_cmd_high,cur_setpoint] =...
    code_gen_grip(delta,max_pos,prev_setpoint)

% Add offset
%motor_1_cmd  = uint16(abs(pos_setpoint));
if( delta >= 200.0 )
    motor_1_cmd  = uint16(abs(max_pos));
elseif( delta <= -200.0 )
    motor_1_cmd  = uint16(abs(0));
else
    motor_1_cmd = uint16(prev_setpoint)
end

cur_setpoint = double(motor_1_cmd);

%% Prepare motor output
m1_cmd_low = uint8(uint16(192) + bitand(motor_1_cmd, uint16(31)));
m1_cmd_high = uint8(bitand(bitshift(motor_1_cmd, -5), uint16(127)));

end
